simulink model "red_adelanto_ao_ej2_2017"  (R2020b)
settings: Solver=VariableStepAuto  StartTime=0.0  StopTime=18  MaxStep=1e-4  RelTol=1e-3
values from neighbouring files (symbols this model uses):
  K = 1/div    [eje_comp_ade.m]
  p = x2+abs(real(s1))    [eje_comp_ade.m]
  R1 = 10e3    (= 10000)    [eje_comp_ade.m]
  R1c = 1/(z*C1)    [eje_comp_ade.m]
  R2 = R1    (= 10000)    [eje_comp_ade.m]
  R2c = 1/(p*C2)    [eje_comp_ade.m]
  R3 = R1    (= 10000)    [eje_comp_ade.m]
  R3c = 10e3    (= 10000)    [eje_comp_ade.m]
  R4 = R1    (= 10000)    [eje_comp_ade.m]
  R4c = K*R3c    [eje_comp_ade.m]
  wn = 4/(Ts*e)    [eje_comp_ade.m]
  z = abs(real(s1))-x1    [eje_comp_ade.m]
libraries: fl_lib x25, nesl_utility x5, ee_lib x1
settings Model: Creator=cmparedes  LastModifiedBy=Acer
settings DataIOCC: ReturnWorkspaceOutputs=off
settings DebuggingCC: ArithmeticOperatorsInVariantConditions=warning
settings SFSimCC: SimUseLocalCustomCode=off  CustomCodeUndefinedFunction=UseInterfaceOnly
settings RTWCC: RTWUseLocalCustomCode=off
settings CodeAppCC: StateflowObjectComments=on

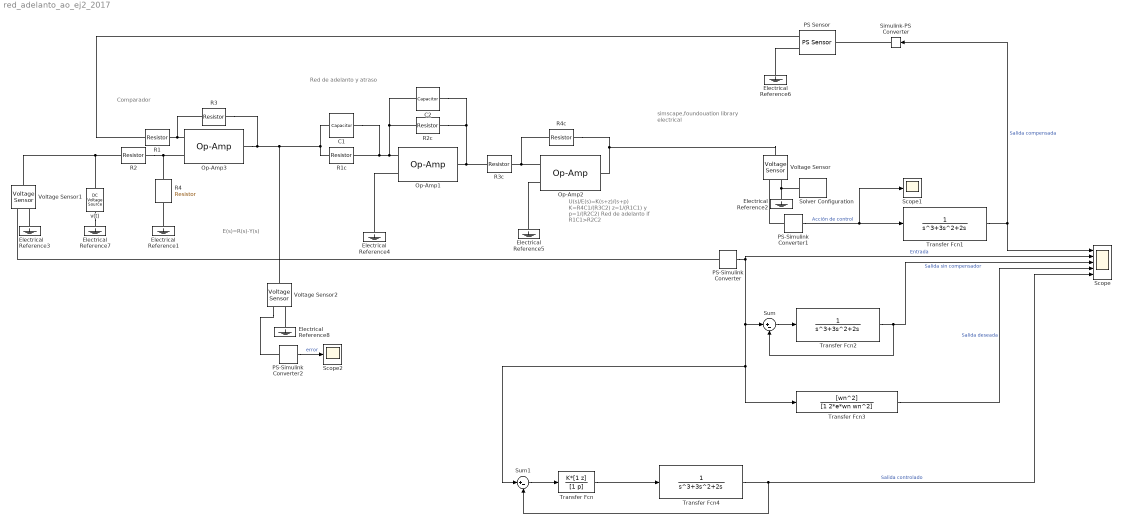
== system red_adelanto_ao_ej2_2017 ==
  note: Red de adelanto y atraso
  note: E(s)=R(s)-Y(s)
  note: Comparador
  note: simscape,foundouation library electrical
  note: U(s)/E(s)=K(s+z)/(s+p)
      |
      | K=R4C1/(R3C2)
      | z=1/(R1C1)  y p=1/(R2C2)
      |
      | Red de adelanto if R1C1>R2C2
  C1 : fl_lib/Electrical/Electrical Elements/Capacitor  c=C1 F  r=1e-6 Ohm  g=0 1/Ohm  i_specify=off  i_priority=None  i=0 A  i_nominal_specify=off  i_nominal_unit=A  i_nominal_value=1  v_specify=off  v_priority=None  v=0 V  v_nominal_specify=off  v_nominal_unit=V  v_nominal_value=1  vc_specify=off  vc_priority=High  vc=0 V  vc_nominal_specify=off  vc_nominal_unit=V  vc_nominal_value=1
  C2 : fl_lib/Electrical/Electrical Elements/Capacitor  c=C2 F  r=1e-6 Ohm  g=0 1/Ohm  i_specify=off  i_priority=None  i=0 A  i_nominal_specify=off  i_nominal_unit=A  i_nominal_value=1  v_specify=off  v_priority=None  v=0 V  v_nominal_specify=off  v_nominal_unit=V  v_nominal_value=1  vc_specify=off  vc_priority=High  vc=0 V  vc_nominal_specify=off  vc_nominal_unit=V  vc_nominal_value=1
  Electrical Reference{1..8} (8 alike) : fl_lib/Electrical/Electrical Elements/Electrical Reference
  Op-Amp1 : fl_lib/Electrical/Electrical Elements/Op-Amp  outI_specify=off  outI_priority=None  outI=0 A  outI_nominal_specify=off  outI_nominal_unit=A  outI_nominal_value=1
  Op-Amp2 : fl_lib/Electrical/Electrical Elements/Op-Amp  outI_specify=off  outI_priority=None  outI=0 A  outI_nominal_specify=off  outI_nominal_unit=A  outI_nominal_value=1
  Op-Amp3 : fl_lib/Electrical/Electrical Elements/Op-Amp  outI_specify=off  outI_priority=None  outI=0 A  outI_nominal_specify=off  outI_nominal_unit=A  outI_nominal_value=1
  PS Sensor : ee_lib/Sensors & Transducers/PS Sensor  op_type=1  A=1  B=0  Ymax=inf  Ymin=-inf
      settings: SourceProductBaseCode=PS  InternalSimscapePortConfiguration="{\"Bottom\":[],\"Left\":[{\"id\":\"U\",\"label\":\"U\",\"type\":\"input\"}],\"Right\":[{\"id\":\"p\",\"label\":\"+\",\"type\":\"foundation.electrical.electrical\"},{\"id\":\"n\",\"label\":\"-\",\"type\":\"foundation.electrical.electrical\"}],\"Top\":[]}"
  PS-Simulink Converter : nesl_utility/PS-Simulink Converter  PhysicalDomain=network_engine_domain  SubClassName=ps_output  LeftPortType=input  RightPortType=output  PseudoPeriodic=off  Frequencies=[]  Unit=1  AffineConversion=off
  PS-Simulink Converter1 : nesl_utility/PS-Simulink Converter  PhysicalDomain=network_engine_domain  SubClassName=ps_output  LeftPortType=input  RightPortType=output  PseudoPeriodic=off  Frequencies=[]  Unit=1  AffineConversion=off
  PS-Simulink Converter2 : nesl_utility/PS-Simulink Converter  PhysicalDomain=network_engine_domain  SubClassName=ps_output  LeftPortType=input  RightPortType=output  PseudoPeriodic=off  Frequencies=[]  Unit=1  AffineConversion=off
  R1 : fl_lib/Electrical/Electrical Elements/Resistor  R=R1 Ohm  i_specify=off  i_priority=None  i=0 A  i_nominal_specify=off  i_nominal_unit=A  i_nominal_value=1  v_specify=off  v_priority=None  v=0 V  v_nominal_specify=off  v_nominal_unit=V  v_nominal_value=1
  R1c : fl_lib/Electrical/Electrical Elements/Resistor  R=R1c Ohm  i_specify=off  i_priority=None  i=0 A  i_nominal_specify=off  i_nominal_unit=A  i_nominal_value=1  v_specify=off  v_priority=None  v=0 V  v_nominal_specify=off  v_nominal_unit=V  v_nominal_value=1
  R2 : fl_lib/Electrical/Electrical Elements/Resistor  R=R2 Ohm  i_specify=off  i_priority=None  i=0 A  i_nominal_specify=off  i_nominal_unit=A  i_nominal_value=1  v_specify=off  v_priority=None  v=0 V  v_nominal_specify=off  v_nominal_unit=V  v_nominal_value=1
  R2c : fl_lib/Electrical/Electrical Elements/Resistor  R=R2c Ohm  i_specify=off  i_priority=None  i=0 A  i_nominal_specify=off  i_nominal_unit=A  i_nominal_value=1  v_specify=off  v_priority=None  v=0 V  v_nominal_specify=off  v_nominal_unit=V  v_nominal_value=1
  R3 : fl_lib/Electrical/Electrical Elements/Resistor  R=R3 Ohm  i_specify=off  i_priority=None  i=0 A  i_nominal_specify=off  i_nominal_unit=A  i_nominal_value=1  v_specify=off  v_priority=None  v=0 V  v_nominal_specify=off  v_nominal_unit=V  v_nominal_value=1
  R3c : fl_lib/Electrical/Electrical Elements/Resistor  R=R3c Ohm  i_specify=off  i_priority=None  i=0 A  i_nominal_specify=off  i_nominal_unit=A  i_nominal_value=1  v_specify=off  v_priority=None  v=0 V  v_nominal_specify=off  v_nominal_unit=V  v_nominal_value=1
  R4 : fl_lib/Electrical/Electrical Elements/Resistor  R=R4 Ohm  i_specify=off  i_priority=None  i=0 A  i_nominal_specify=off  i_nominal_unit=A  i_nominal_value=1  v_specify=off  v_priority=None  v=0 V  v_nominal_specify=off  v_nominal_unit=V  v_nominal_value=1
  R4c : fl_lib/Electrical/Electrical Elements/Resistor  R=R4c Ohm  i_specify=off  i_priority=None  i=0 A  i_nominal_specify=off  i_nominal_unit=A  i_nominal_value=1  v_specify=off  v_priority=None  v=0 V  v_nominal_specify=off  v_nominal_unit=V  v_nominal_value=1
  Scope : Scope  NumInputPorts=5
  Scope1 : Scope
  Scope2 : Scope
  Simulink-PS Converter : nesl_utility/Simulink-PS Converter  PhysicalDomain=network_engine_domain  SubClassName=ps_input  LeftPortType=input  RightPortType=output  PseudoPeriodic=off  Frequencies=[]  NoiseDistribution=none  NoiseParameters=[]  Unit=1  AffineConversion=off  FilteringAndDerivatives=provide  SimscapeFilterOrder=1  InputFilterTimeConstant=0.001  UdotUserProvided=0
  Solver Configuration : nesl_utility/Solver Configuration  PhysicalDomain=network_engine_domain  SubClassName=solver  LeftPortType=input  RightPortType=generic  Tones=[]  Harmonics=[]  SimulateNoise=off  Profile=off  UseLocalSampling=off  EnableSwitchedLinearOptims=on  FrequencyDomain=off  UseCCode=off  RelTol=0.001  AbsTol=1e-06  MinStep=1e-09  ToWorkspace=off  RevertToSquareIcSolve=off  NumHomotopyIterations=100  PhasorMode=off  PhasorModeNumHarmonics=1  DoDC=off  ResidualTolerance=1e-09  UseLocalSolver=off  LocalSolverChoice=NE_BACKWARD_EULER_ADVANCER  LocalSolverSampleTime=0.001  DoFixedCost=off  MaxNonlinIter=3  MaxModeIter=2  ComputeImpulses=off  ImpulseIterations=2  LinearAlgebra=Sparse  EquationFormulation=NE_TIME_EF  DelaysMemoryBudget=1024  AutomaticFiltering=on  FilteringTimeConstant=0.001  PartitionStorageMethod=AS_NEEDED  PartitionMemoryBudget=1024  PartitionMethod=FAST
  Sum : Sum  Inputs=|+-
  Sum1 : Sum  Inputs=|+-
  Transfer Fcn : TransferFcn  Numerator=K*[1 z]  Denominator=[1 p]
  Transfer Fcn1 : TransferFcn  Denominator=[1 3 2 0]
  Transfer Fcn2 : TransferFcn  Denominator=[1 3 2 0]
  Transfer Fcn3 : TransferFcn  Numerator=[wn^2]  Denominator=[1 2*e*wn wn^2]
  Transfer Fcn4 : TransferFcn  Denominator=[1 3 2 0]
  Voltage Sensor : fl_lib/Electrical/Electrical Sensors/Voltage Sensor
  Voltage Sensor1 : fl_lib/Electrical/Electrical Sensors/Voltage Sensor
  Voltage Sensor2 : fl_lib/Electrical/Electrical Sensors/Voltage Sensor
  v(t) : fl_lib/Electrical/Electrical Sources/DC Voltage Source  v0=1 V
  wires:
  PS-Simulink Converter1/1 -> Transfer Fcn1/1, Scope1/1  "Acción de control"
  Transfer Fcn1/1 -> Simulink-PS Converter/1, Scope/1  "Salida compensada"
  Sum/1 -> Transfer Fcn2/1
  Transfer Fcn2/1 -> Scope/3, Sum/2  "Salida sin compensador"
  Transfer Fcn3/1 -> Scope/4  "Salida deseada"
  PS-Simulink Converter2/1 -> Scope2/1  "error"
  Transfer Fcn4/1 -> Scope/5, Sum1/2  "Salida controlado"
  PS-Simulink Converter/1 -> Sum1/1, Transfer Fcn3/1, Sum/1, Scope/2  "Entrada"
  Sum1/1 -> Transfer Fcn/1
  Transfer Fcn/1 -> Transfer Fcn4/1
  connections:
  Electrical Reference2/LConn1 -- Solver Configuration/RConn1 -- Voltage Sensor/RConn2
  PS-Simulink Converter1/LConn1 -- Voltage Sensor/RConn1
  PS-Simulink Converter/LConn1 -- Voltage Sensor1/RConn1
  R2/RConn1 -- R4/RConn1 -- Op-Amp3/LConn1
  Electrical Reference1/LConn1 -- R4/LConn1
  R1/RConn1 -- R3/LConn1 -- Op-Amp3/LConn2
  Voltage Sensor1/LConn1 -- v(t)/LConn1 -- R2/LConn1
  Electrical Reference3/LConn1 -- Voltage Sensor1/RConn2
  Op-Amp1/LConn2 -- C2/LConn1 -- R2c/LConn1 -- C1/RConn1 -- R1c/RConn1
  R2c/RConn1 -- C2/RConn1 -- R3c/LConn1 -- Op-Amp1/RConn1
  Electrical Reference4/LConn1 -- Op-Amp1/LConn1
  C1/LConn1 -- Voltage Sensor2/LConn1 -- R3/RConn1 -- Op-Amp3/RConn1 -- R1c/LConn1
  R3c/RConn1 -- R4c/LConn1 -- Op-Amp2/LConn2
  R4c/RConn1 -- Voltage Sensor/LConn1 -- Op-Amp2/RConn1
  Electrical Reference5/LConn1 -- Op-Amp2/LConn1
  PS Sensor/RConn1 -- R1/LConn1
  Simulink-PS Converter/RConn1 -- PS Sensor/LConn1
  PS Sensor/RConn2 -- Electrical Reference6/LConn1
  v(t)/RConn1 -- Electrical Reference7/LConn1
  Electrical Reference8/LConn1 -- Voltage Sensor2/RConn2
  Voltage Sensor2/RConn1 -- PS-Simulink Converter2/LConn1
